simulink model "draft6"  (R2023a)
settings: Solver=VariableStepAuto  StartTime=0.0  StopTime=1  FixedStep=0.0001  MaxStep=0.2  RelTol=1e-3  AbsTol=1e-3  EnableMultiTasking=on
model workspace (MAT data in the model file):
  LeftAbdominalMuscleForce = -90
  LeftBackMuscleForce = 0
  LeftTransverseMucleForce1 = 0
  LeftTransverseMuscleForce2 = 0
  RightAbdominalMuscleForce = -90
  RightBackMuscleForce = 0
  RightTransverseMuscleForce1 = 0
  RightTransverseMuscleForce2 = 0
  c = 0.1
  k : Simulink.Parameter (value not decoded)
libraries: nesl_utility x47, sm_lib x25, simulink_extras x3, checkpacklib x1
(part 3 of 3)

== matlab function draft6/L1/FE torque feedback L4/peacewise torque profile1 ==
  data: u input; torque output
function torque = T(u)
torque = 0;
if (u >= 15)
    torque= -0.0015*1*(57.295*15)^4 + 0.1326*(57.295*15)^3 -0.3477*(57.295*15)^2 + 0.499*(57.295*15);
 
elseif (u >= -15 && u<= 15)
    torque= -0.0015*(57.295*u)^4 + 0.1326*(57.295*u)^3 -0.3477*(57.295*u)^2 + 0.499*(57.295*u)   ;
    
elseif (u <= -15)
   torque= -0.0015*1*(57.295*-15)^4 + 0.1326*(57.295*-15)^3 -0.3477*(57.295*-15)^2 + 0.499*(57.295*-15);
end
